simulink model "system_model_script_interactive"  (R2013a)
settings: Solver=ode15s  StartTime=0.0  StopTime=10  FixedStep=.1  MaxStep=0.001  RelTol=1e-3
values from neighbouring files (symbols this model uses):
  Ga = 3    [a2_data_input_examsim1.m]    (also in a2_data_input_examsim2.m = 1; a2_data_input_hw3.m = 0.095; a2_data_input_mdcs_h5_v1_stud_p1.m = 0.095; a2_data_input_mdcs_h5_v1_stud_p4.m = 0.006)
  Gf = Gr/(Kd*Gs)    [a3_process_input.m]
  Gs = 1    [a2_data_input_examsim1.m]    (also in a2_data_input_examsim2.m = 5; a2_data_input_hw3.m; a2_data_input_mdcs_h5_v1_stud_p1.m; a2_data_input_mdcs_h5_v1_stud_p4.m)
  Kd = 2    [a2_data_input_examsim1.m]    (also in a2_data_input_examsim2.m = 1; a2_data_input_hw3.m = 1; a2_data_input_mdcs_h5_v1_stud_p1.m = 1; a2_data_input_mdcs_h5_v1_stud_p4.m = 1)
undefined symbols (not defined in the file or in its folder): da, dp, ds, r
libraries: cstblocks x6
settings Model: Creator=s177063  LastModifiedBy=s171105
settings DataIOCC: ExternalInput=[t,u]  LimitDataPoints=off  LoadExternalInput=on  SaveOutput=off  SignalLogging=off
settings OptimizationCC: ExpressionDepthLimit=2147483647
settings GRTTargetCC: CombineOutputUpdateFcns=off  GRTInterface=on

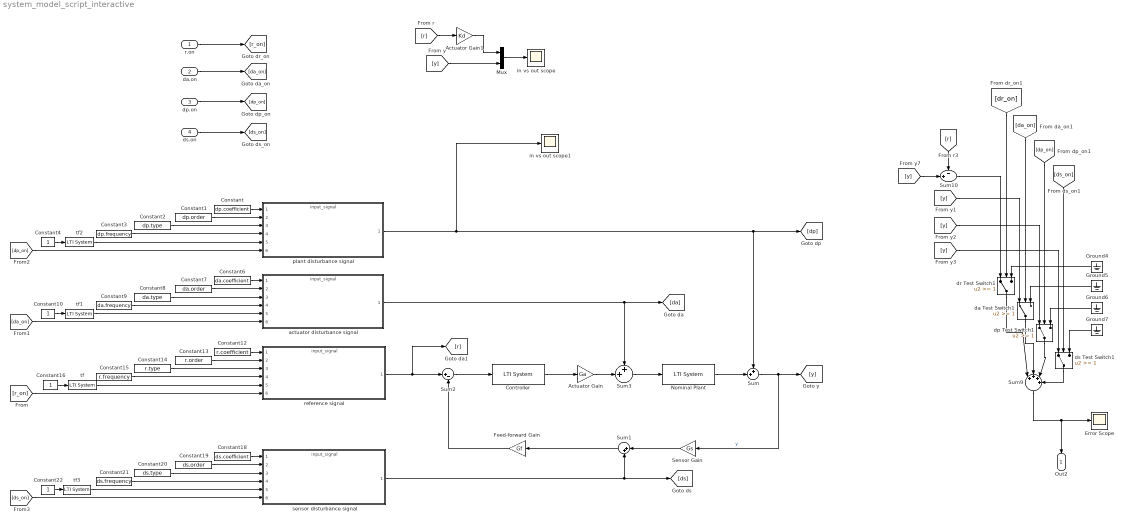
== system system_model_script_interactive ==
  r.on : Inport
  da.on : Inport  Port=2
  dp.on : Inport  Port=3
  ds.on : Inport  Port=4
  Actuator Gain : Gain  Gain=Ga
  Actuator Gain1 : Gain  Gain=Kd
  Constant : Constant  Value=dp.coefficient
  Constant1 : Constant  Value=dp.order
  Constant{4,10,16,22} (4 alike) : Constant
  Constant12 : Constant  Value=r.coefficient
  Constant13 : Constant  Value=r.order
  Constant14 : Constant  Value=r.type
  Constant15 : Constant  Value=r.frequency
  Constant18 : Constant  Value=ds.coefficient
  Constant19 : Constant  Value=ds.order
  Constant2 : Constant  Value=dp.type
  Constant20 : Constant  Value=ds.type
  Constant21 : Constant  Value=ds.frequency
  Constant3 : Constant  Value=dp.frequency
  Constant6 : Constant  Value=da.coefficient
  Constant7 : Constant  Value=da.order
  Constant8 : Constant  Value=da.type
  Constant9 : Constant  Value=da.frequency
  Controller : cstblocks/LTI System  sys=Gc.mod.value  IC=[]
  Error Scope : Scope
      settings: TimeRange=0.5  YMin=0  YMax=2.5  SampleInput=on
  Feed-forward Gain : Gain  Gain=Gf
  Ground{4..7} (4 alike) : Ground
  Mux : Mux  Inputs=2
  Nominal Plant : cstblocks/LTI System  sys=Gp.nominal.tf  IC=[]
  Sensor Gain : Gain  Gain=Gs
  Sum : Sum  Inputs=++|
  Sum1 : Sum  Inputs=|++
  Sum10 : Sum  Inputs=-+|
  Sum2 : Sum  Inputs=|+-
  Sum3 : Sum  Inputs=++|
  Sum9 : Sum  Inputs=|++++
  actuator disturbance signal : ModelReference  ModelNameDialog=input_signal  ModelReferenceVersion=1.18  CopyOfModelName=input_signal  DefaultDataLogging=off
  da Test Switch1 : Switch  Threshold=1
  dp Test Switch1 : Switch  Threshold=1
  dr Test Switch1 : Switch  Threshold=1
  ds Test Switch1 : Switch  Threshold=1
  in vs out scope : Scope
      settings: TimeRange=0.5  YMin=7.45  YMax=8.3  SampleInput=on
  in vs out scope1 : Scope
      settings: TimeRange=0.5  YMin=-1  YMax=1  SaveName=ScopeData2  SampleInput=on
  plant disturbance signal : ModelReference  ModelNameDialog=input_signal  ModelReferenceVersion=1.18  CopyOfModelName=input_signal  DefaultDataLogging=off
  reference signal : ModelReference  ModelNameDialog=input_signal  ModelReferenceVersion=1.18  CopyOfModelName=input_signal  DefaultDataLogging=off
  sensor disturbance signal : ModelReference  ModelNameDialog=input_signal  ModelReferenceVersion=1.18  CopyOfModelName=input_signal  DefaultDataLogging=off
  tf : cstblocks/LTI System  sys=r.tf  IC=[]
  tf1 : cstblocks/LTI System  sys=da.tf  IC=[]
  tf2 : cstblocks/LTI System  sys=dp.tf  IC=[]
  tf3 : cstblocks/LTI System  sys=ds.tf  IC=[]
  Out2 : Outport
  wires:
  Sum/1 -> Sensor Gain/1, [y]  "y"
  Controller/1 -> Actuator Gain/1
  Sum3/1 -> Nominal Plant/1
  Sum2/1 -> Controller/1
  Sensor Gain/1 -> Sum1/1
  Sum1/1 -> Feed-forward Gain/1
  Feed-forward Gain/1 -> Sum2/2
  Actuator Gain/1 -> Sum3/2
  Nominal Plant/1 -> Sum/2
  reference signal/1 -> Sum2/1, [r]
  actuator disturbance signal/1 -> Sum3/1, [da]
  plant disturbance signal/1 -> Sum/1, [dp], in vs out scope1/1
  sensor disturbance signal/1 -> Sum1/2, [ds]
  Constant/1 -> plant disturbance signal/1
  Constant1/1 -> plant disturbance signal/2
  Constant2/1 -> plant disturbance signal/3
  Constant3/1 -> plant disturbance signal/4
  tf2/1 -> plant disturbance signal/5
  Constant6/1 -> actuator disturbance signal/1
  Constant7/1 -> actuator disturbance signal/2
  Constant8/1 -> actuator disturbance signal/3
  Constant9/1 -> actuator disturbance signal/4
  tf1/1 -> actuator disturbance signal/5
  [da_on] -> actuator disturbance signal/6
  Constant12/1 -> reference signal/1
  Constant13/1 -> reference signal/2
  Constant14/1 -> reference signal/3
  Constant15/1 -> reference signal/4
  tf/1 -> reference signal/5
  [r_on] -> reference signal/6
  Constant18/1 -> sensor disturbance signal/1
  Constant19/1 -> sensor disturbance signal/2
  Constant20/1 -> sensor disturbance signal/3
  Constant21/1 -> sensor disturbance signal/4
  tf3/1 -> sensor disturbance signal/5
  [ds_on] -> sensor disturbance signal/6
  Constant16/1 -> tf/1
  Constant10/1 -> tf1/1
  Constant4/1 -> tf2/1
  Constant22/1 -> tf3/1
  r.on/1 -> [r_on]
  da.on/1 -> [da_on]
  dp.on/1 -> [dp_on]
  ds.on/1 -> [ds_on]
  [dp_on] -> plant disturbance signal/6
  Mux/1 -> in vs out scope/1
  Sum10/1 -> dr Test Switch1/1
  [y] -> da Test Switch1/1
  [y] -> dp Test Switch1/1
  [y] -> ds Test Switch1/1
  [dr_on] -> dr Test Switch1/2
  [da_on] -> da Test Switch1/2
  [dp_on] -> dp Test Switch1/2
  [ds_on] -> ds Test Switch1/2
  dr Test Switch1/1 -> Sum9/1
  da Test Switch1/1 -> Sum9/2
  dp Test Switch1/1 -> Sum9/3
  ds Test Switch1/1 -> Sum9/4
  Ground4/1 -> dr Test Switch1/3
  Ground5/1 -> da Test Switch1/3
  Ground6/1 -> dp Test Switch1/3
  Ground7/1 -> ds Test Switch1/3
  [r] -> Sum10/1
  [y] -> Sum10/2
  Sum9/1 -> Error Scope/1, Out2/1
  [r] -> Actuator Gain1/1
  Actuator Gain1/1 -> Mux/1
  [y] -> Mux/2
